simulink model "backstepping_compliant_two_motors"  (R2022b)
settings: Solver=VariableStepAuto  StartTime=0.0  StopTime=20  RelTol=1e-3
values from neighbouring files (symbols this model uses):
  Lamda = 1*eye(2)    [init.m]
undefined symbols (not defined in the file or in its folder): D, J
settings Model: Creator=alexi  LastModifiedBy=alexi

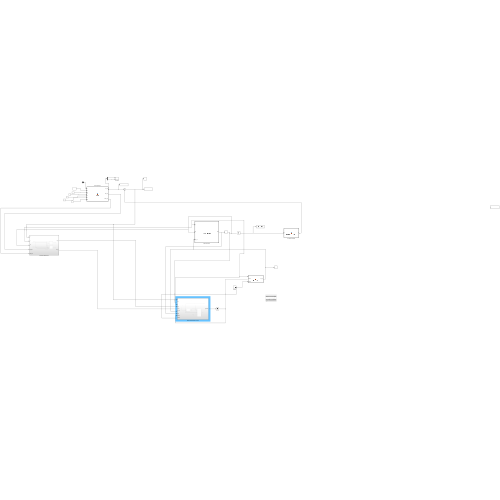
[thumbnail: Simulink's stored preview of the top-level diagram]
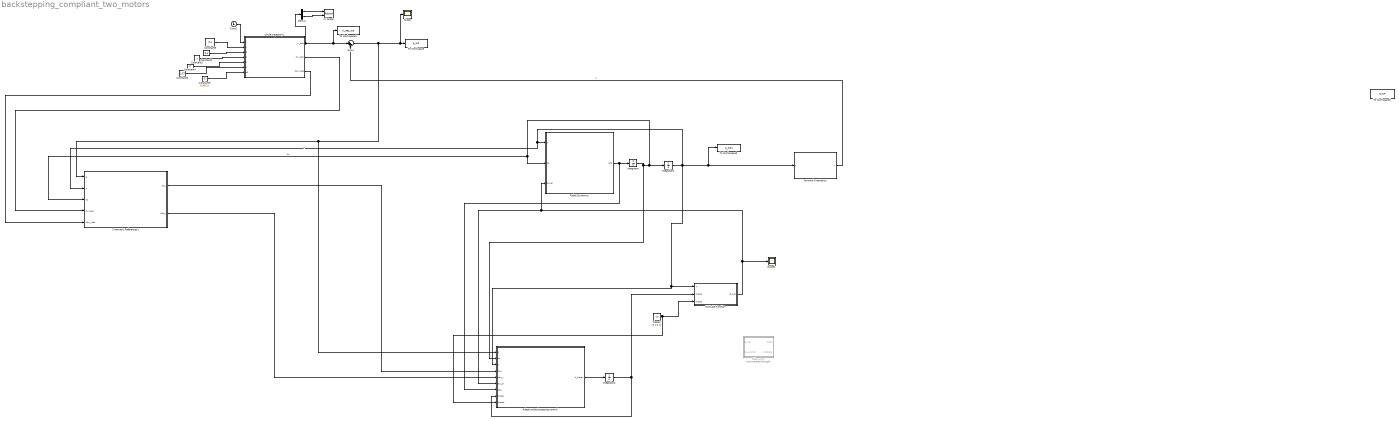
== system backstepping_compliant_two_motors ==
  Adaptive Backstepping control : Subsystem
  Clock1 : Clock
  Constant2 : Constant  Value=0.4
  Constant3 : Constant
  Constant4 : Constant  Value=2
  Constant5 : Constant  Value=1.57
  Constant6 : Constant  Value=[0.85,1]
  Constant9 : Constant  Value=0.4
  Demux : Demux  Outputs=2
  Forward Kinematics : MATLAB Function  TreatAsAtomicUnit=on
  Integrator : Integrator  InitialCondition=[0,0]'
  Integrator1 : Integrator  InitialCondition=[0.1,0.1]'
  Integrator2 : Integrator  InitialCondition=[0.1,0.1]'
  Kinematic References1 : Subsystem
  MATLAB Function : MATLAB Function  TreatAsAtomicUnit=on
  Robot Dynamics : MATLAB Function  TreatAsAtomicUnit=on
  Scope : Scope
  Scope1 : Scope
  Subsystem : Subsystem  Commented=through
  Sum4 : Sum  Inputs=|+-
  To Workspace : ToWorkspace  VariableName=e_out  SaveFormat=Timeseries  SampleTime=-1
  To Workspace1 : ToWorkspace  VariableName=xi_des_out  SaveFormat=Timeseries  SampleTime=-1
  To Workspace2 : ToWorkspace  VariableName=q_out  SaveFormat=Timeseries  SampleTime=-1
  To Workspace3 : ToWorkspace  VariableName=q_out1  SaveFormat=Timeseries  SampleTime=-1
  XY Graph : Record  FileSettingsInternal="{\"entries\":[{\"content\":{\"excelSettings\":{\"content\":{},\"type\":\"Streamout.ExcelSettings\"}},\"type\":\"Streamout.FileSettingStorage\",\"uuid\":\"296eadd8-438a-48ea-aa87-085f53f925dc\"}],\"packageUris\":[\"http://schema.mathworks.com/mf0/streamout_blocks/R2020a\"],\"version\":\"1.0\"}"  Layout=[1 1]  SignalsInternal="{\"entries\":[{\"content\":{\"signals\":[{\"content\":{\"blockPath\":[\"backstepping_compliant_two_motors/XY Graph\"],\"channel\":[],\"dimensions\":[1],\"domain\":\"backstepping_compliant_two_motors/XY Graph\",\"lineColor\":\"#a2142f\",\"plots\":[],\"port\":1,\"sid\":[\"\"],\"signalID\":2831,\"signalName\":\"Demux:1\"},\"type\":\"RecordBlkView.Signal\",\"uuid\":\"da436bb7-b6f0-4922-b408-d20702b7c22f\"},{\"content\":{\"blockPath\":[\"backstepping_compliant_two_motors/XY Graph\"],\"channel\":[],\"dimensions\":[1],\"domain\":\"backstepping_compliant_two_motors/XY Graph\",\"lineColor\":\"#139fff\",\"plots\":[],\"port\":2,\"sid\":[\"\"],\"signalID\":2835,\"signalName\":\"Demux:2\"},\"type\":\"RecordBlkView.Signal\",\"uuid\":\"9bd5da55-d73b-4537-9ebd-c9d85c402df8\"}]},\"type\":\"RecordBlkView.InputSignals\",\"uuid\":\"734fe5a4-c58d-4aeb-987a-d06effc65ad3\"}],\"packageUris\":[\"http://schema.mathworks.com/mf0/streamout_blocks/R2020a\"],\"version\":\"1.0\"}"  VisualizationBindings="{\"xyplotplugin\":{\"info\":[{\"series\":[],\"subplotID\":1}]}}"  CompatibilityTag=XY
  circle trajectory1 : MATLAB Function  TreatAsAtomicUnit=on
  thetad : Constant  Value=[0.1,0.1]'
  wires:
  Clock1/1 -> circle trajectory1/1(t)
  Constant9/1 -> circle trajectory1/2(A)
  Constant2/1 -> circle trajectory1/3(B)
  Constant3/1 -> circle trajectory1/4(a)
  Constant4/1 -> circle trajectory1/5(b)
  Constant5/1 -> circle trajectory1/6(d)
  Constant6/1 -> circle trajectory1/7(p0)
  Integrator/1 -> Adaptive Backstepping control/2(dq), Integrator1/1, Robot Dynamics/2(dq), Kinematic References1/3(dq)  "dq"
  Robot Dynamics/1(ddq) -> Adaptive Backstepping control/7(ddq), Integrator/1
  Integrator1/1 -> Adaptive Backstepping control/3(q), MATLAB Function/1(q), Forward Kinematics/1(q), To Workspace3/1, Kinematic References1/2(q), Robot Dynamics/1(q)  "q"
  circle trajectory1/1(xi_des) -> Demux/1, To Workspace1/1, Sum4/1
  Forward Kinematics/1(xi) -> Sum4/2  "xi"
  Sum4/1 -> Scope/1, To Workspace/1, Adaptive Backstepping control/1(e), Kinematic References1/1(e)
  circle trajectory1/2(dxi_des) -> Kinematic References1/4(dxi_des)
  Kinematic References1/1(dq_r) -> Adaptive Backstepping control/4(dq_r)
  Kinematic References1/2(ddq_r) -> Adaptive Backstepping control/5(ddq_r)
  Adaptive Backstepping control/1(d_thetas) -> Integrator2/1
  Integrator2/1 -> Adaptive Backstepping control/8(thetas), MATLAB Function/2(thetas)
  MATLAB Function/1(tau_el) -> Scope1/1, Robot Dynamics/3(tau_el), Adaptive Backstepping control/6(tau_el)
  circle trajectory1/3(ddxi_des) -> Kinematic References1/5(ddxi_des)
  Demux/1 -> XY Graph/1
  Demux/2 -> XY Graph/2
  thetad/1 -> Adaptive Backstepping control/9(thetad), MATLAB Function/3(thetad)

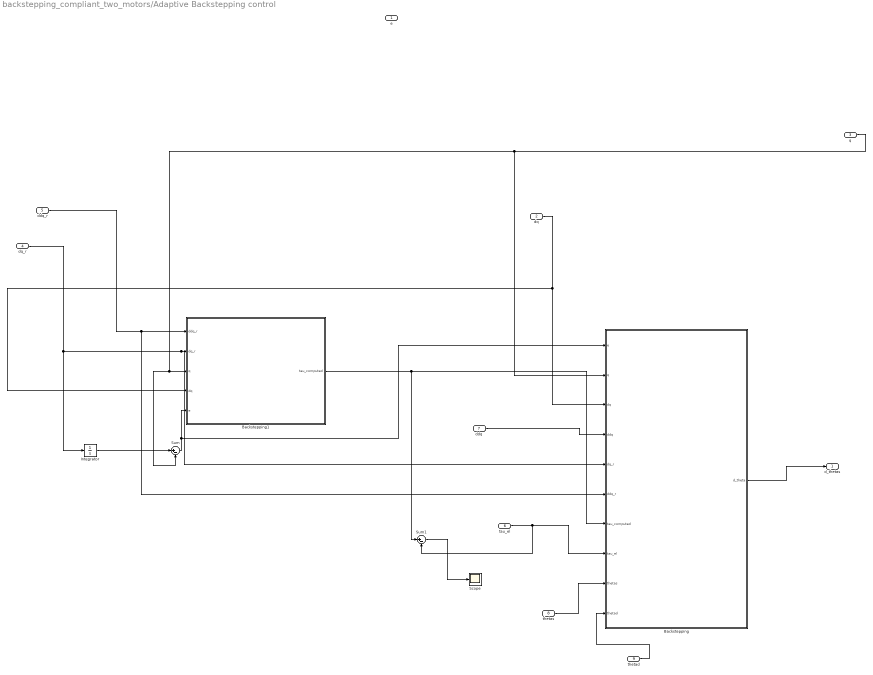
== system backstepping_compliant_two_motors/Adaptive Backstepping control ==
  e : Inport
  dq : Inport  Port=2
  q : Inport  Port=3
  dq_r : Inport  Port=4
  ddq_r : Inport  Port=5
  tau_el : Inport  Port=6
  ddq : Inport  Port=7
  thetas : Inport  Port=8
  thetad : Inport  Port=9
  Backstepping : MATLAB Function  TreatAsAtomicUnit=on
  Backstepping1 : MATLAB Function  TreatAsAtomicUnit=on
  Integrator : Integrator  InitialCondition=[0.1,0.1]'
  Scope : Scope
  Sum : Sum  Inputs=|+-
  Sum1 : Sum  Inputs=|+-
  d_thetas : Outport
  wires:
  dq_r/1 -> Integrator/1, Backstepping1/2(dq_r), Backstepping/5(dq_r)
  q/1 -> Backstepping/2(q), Backstepping1/3(q), Sum/2
  Backstepping1/1(tau_computed) -> Sum1/1, Backstepping/7(tau_computed)
  tau_el/1 -> Sum1/2, Backstepping/8(tau_el)
  ddq_r/1 -> Backstepping/6(ddq_r), Backstepping1/1(ddq_r)
  dq/1 -> Backstepping1/4(dq), Backstepping/3(dq)
  Backstepping/1(d_theta) -> d_thetas/1
  ddq/1 -> Backstepping/4(ddq)
  thetas/1 -> Backstepping/9(thetas)
  Integrator/1 -> Sum/1
  Sum/1 -> Backstepping1/5(e), Backstepping/1(e)
  thetad/1 -> Backstepping/10(thetad)
  Sum1/1 -> Scope/1

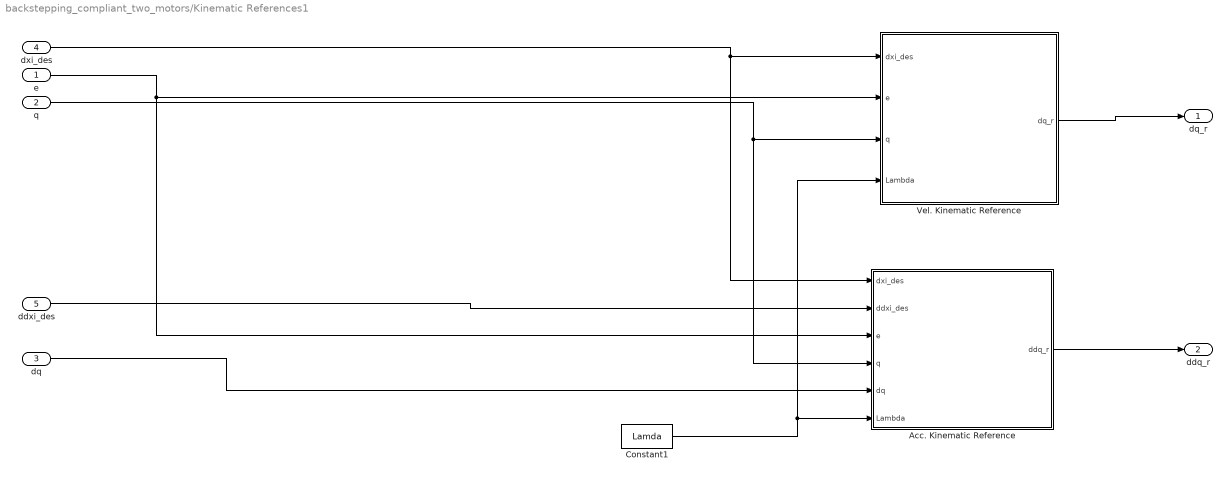
== system backstepping_compliant_two_motors/Kinematic References1 ==
  e : Inport
  q : Inport  Port=2
  dq : Inport  Port=3
  dxi_des : Inport  Port=4
  ddxi_des : Inport  Port=5
  Acc. Kinematic Reference : MATLAB Function  TreatAsAtomicUnit=on
  Constant1 : Constant  Value=Lamda
  "Vel. Kinematic Reference " : MATLAB Function  TreatAsAtomicUnit=on
  dq_r : Outport  VectorParamsAs1DForOutWhenUnconnected=off
  ddq_r : Outport  Port=2  VectorParamsAs1DForOutWhenUnconnected=off
  wires:
  ddxi_des/1 -> Acc. Kinematic Reference/2(ddxi_des)
  e/1 -> Acc. Kinematic Reference/3(e), "Vel. Kinematic Reference "/2(e)
  dxi_des/1 -> Acc. Kinematic Reference/1(dxi_des), "Vel. Kinematic Reference "/1(dxi_des)
  Constant1/1 -> "Vel. Kinematic Reference "/4(Lambda), Acc. Kinematic Reference/6(Lambda)
  "Vel. Kinematic Reference "/1(dq_r) -> dq_r/1
  dq/1 -> Acc. Kinematic Reference/5(dq)
  q/1 -> Acc. Kinematic Reference/4(q), "Vel. Kinematic Reference "/3(q)
  Acc. Kinematic Reference/1(ddq_r) -> ddq_r/1

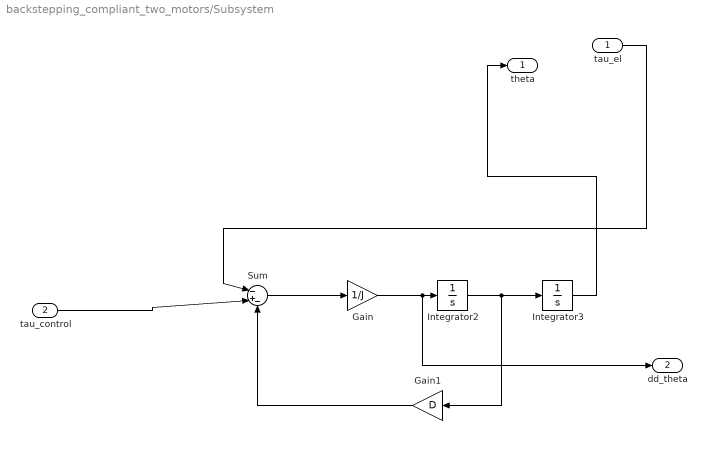
== system backstepping_compliant_two_motors/Subsystem ==
  tau_el : Inport
  tau_control : Inport  Port=2
  Gain : Gain  Gain=1/J
  Gain1 : Gain  Gain=D
  Integrator2 : Integrator
  Integrator3 : Integrator
  Sum : Sum  Inputs=|-+-
  theta : Outport
  dd_theta : Outport  Port=2
  wires:
  tau_control/1 -> Sum/2
  Integrator3/1 -> theta/1
  Integrator2/1 -> Gain1/1, Integrator3/1
  Gain1/1 -> Sum/3
  Gain/1 -> dd_theta/1, Integrator2/1
  Sum/1 -> Gain/1
  tau_el/1 -> Sum/1

== matlab function backstepping_compliant_two_motors/Kinematic References1/Acc. Kinematic Reference ==
  data: dxi_des input; ddq_r output; ddxi_des input; e input; q input; dq input; Lambda input
function ddq_r = acc_kinematic_reference(dxi_des, ddxi_des, e, q, dq, Lambda)

coder.extrinsic('disp');

J = zeros(2,2);
dJ = zeros(2,2);

dq1 = dq(1);
dq2 = dq(2);

q1 = q(1);
q2 = q(2);

a1 = 1;
a2 = 1;

% Computing jacobian and derivative
J = [-a2*sin(q1 + q2) - a1*sin(q1), -a2*sin(q1 + q2);
      a2*cos(q1 + q2) + a1*cos(q1),  a2*cos(q1 + q2)];

dJ = [-a2*cos(q1 + q2)*(dq1 + dq2)-a1*cos(q1)*dq1, -a2*cos(q1 + q2)*(dq1 + dq2);
    -a2*sin(q1 + q2)*(dq1 + dq2)-a1*sin(q1)*dq1, -a2*sin(q1 + q2)*(dq1 + dq2)];

ddq_r = inv(J) * (ddxi_des + Lambda*dxi_des - Lambda*J*dq) ...
- inv(J)*dJ*inv(J)*(dxi_des + Lambda*e);
end

== matlab function backstepping_compliant_two_motors/Kinematic References1/Vel. Kinematic Reference  ==
  data: dxi_des input; dq_r output; e input; q input; Lambda input
function dq_r = vel_kinematic_reference(dxi_des, e, q, Lambda)
a1 = 1;
a2 = 1;

q1 = q(1);
q2 = q(2);

% Computing jacobian
J = [-a2*sin(q1 + q2) - a1*sin(q1), -a2*sin(q1 + q2);
      a2*cos(q1 + q2) + a1*cos(q1),  a2*cos(q1 + q2)];

dq_r = inv(J) * (dxi_des + Lambda*e);
end

== matlab function backstepping_compliant_two_motors/Adaptive Backstepping control/Backstepping1 ==
  data: ddq_r input; dq_r input; q input; dq input; e input; tau_computed output
function tau_computed  = computed_torque(ddq_r,dq_r,q,dq,e)

coder.extrinsic('disp');
rel_err = 0;

de = dq_r-dq;
Kp = 35;
Kv = 12;

% Get dynamic matrices
B = RR_mass_matrix(q);
C = RR_coriolis_matrix(q,dq);
G = RR_gravity_vector(q);

% Adding uncertainty
B = B.*(1 + rel_err);
C = C.*(1 + rel_err);
G = G.*(1 + rel_err);

% Control law
tau_computed = -(B*ddq_r+C*dq+G+B*Kp*e+B*Kv*de);

== matlab function backstepping_compliant_two_motors/circle trajectory1 ==
  data: t input; xi_des output; dxi_des output; A input; B input; a input; b input; d input; p0 input; ddxi_des output
function [xi_des, dxi_des, ddxi_des] = lissajous(t,A,B,a,b,d,p0)

xi_des = [A*sin(a*t+d); B*sin(b*t)] + p0;
dxi_des = [A*a*cos(a*t+d); B*b*cos(b*t)];
ddxi_des = [-A*a^2*sin(a*t+d); -B*b^2*sin(b*t)];

== matlab function backstepping_compliant_two_motors/MATLAB Function ==
  data: q input; tau_el output; thetas input; thetad input
function tau_el = tau_elastica(q,thetas,thetad)
% k = 0.1;
% a = 9;
% k1_hat = pi(1);
% k2_hat = pi(2);
% k3_hat = pi(3);
% k4_hat = pi(4);
k1 = 100;
k2 = 100;
k3 = 100;
k4 = 100;

tau_el1 = k1*(q(1)-thetas(1)-thetad(1)) + k1*(q(1) - thetas(1) + thetad(1)) + k2*(q(1)-thetas(1) - thetad(1))^2 + k2*(q(1)-thetas(1) + thetad(1))^2 + k3*(q(1)-thetas(1) - thetad(1))^3 + k3*(q(1)-thetas(1) + thetad(1))^3 + k4*(q(1)-thetas(1) - thetad(1))^4 + k4*(q(1)-thetas(1) + thetad(1))^4;
tau_el2 = k1*(q(2)-thetas(2)-thetad(2)) + k1*(q(2) - thetas(2) + thetad(2)) + k2*(q(2)-thetas(2) - thetad(2))^2 + k2*(q(2)-thetas(2) + thetad(2))^2 + k3*(q(2)-thetas(2) - thetad(2))^3 + k3*(q(2)-thetas(2) + thetad(2))^3 + k4*(q(2)-thetas(2) - thetad(2))^4 + k4*(q(2)-thetas(2) + thetad(2))^4;
tau_el = [tau_el1;tau_el2];

== matlab function backstepping_compliant_two_motors/Adaptive Backstepping control/Backstepping ==
  data: e input; q input; dq input; ddq input; dq_r input; ddq_r input; tau_computed input; d_theta output; tau_el input; thetas input; thetad input
function d_theta  = backstepping(e,q,dq,ddq,dq_r,ddq_r,tau_computed,tau_el,thetas,thetad)

coder.extrinsic('disp');
rel_err = 0;
de = dq_r-dq;
dde = ddq_r-ddq;
P = 10*eye(2);
K = 0.1;
Kc = 100;
Kp = 35;
Kv = 12;
a = 9;
% k1_hat = 50;
% k2_hat = 50;
% k3_hat = 50;
% k4_hat = 50;
k1 = 100;
k2 = 100;
k3 = 100;
k4 = 100;

% Get dynamic matrices
B = RR_mass_matrix(q);
C = RR_coriolis_matrix(q,dq);
G = RR_gravity_vector(q);

% Adding uncertainty
B = B.*(1 + rel_err);
C = C.*(1 + rel_err);
G = G.*(1 + rel_err);
g = [zeros(2,2); pinv(B)];
d_tau = C*dde-B*Kv*dde-B*Kp*de;

a1 = 1;
a2 = 1;



% Control law
%d_theta = B*ddq_r + C*dq_r + G + Ks*de + J.'*e;
Vx1 = [e'*Kp,de'];

l1 = -k1 - k1 - 2*k2*(q(1)-thetas(1)-thetad(1)) - 2*k2*(q(1)-thetas(1) + thetad(1)) - 3*k3*(q(1)-thetas(1)-thetad(1))^2 - 3*k3*(q(1)-thetas(1)+thetad(1))^2 - 4*k4*(q(1)-thetas(1)-thetad(1))^3 - 4*k4*(q(1)-thetas(1)+thetad(1))^3 ;
l2 = -k1 - k1 - 2*k2*(q(2)-thetas(2)-thetad(2)) - 2*k2*(q(2)-thetas(2) + thetad(2)) - 3*k3*(q(2)-thetas(2)-thetad(2))^2 - 3*k3*(q(2)-thetas(2)+thetad(2))^2 - 4*k4*(q(2)-thetas(2)-thetad(2))^3 - 4*k4*(q(2)-thetas(2)+thetad(2))^3;


l = [l1 0; 0 l2];


h1 = k1*dq(1) + k1*dq(1) + 2*k2*(q(1)-thetas(1)-thetad(1))*dq(1) + 2*k2*(q(1)-thetas(1)+thetad(1))*dq(1) + 3*k3*dq(1)*(q(1)-thetas(1)-thetad(1))^2 + 3*k3*dq(1)*(q(1)-thetas(1)+thetad(1))^2 + 4*k4*dq(1)*(q(1)-thetas(1)-thetad(1))^3 + 4*k4*dq(1)*(q(1)-thetas(1)+thetad(1))^3;
h2 = k1*dq(2) + k1*dq(2) + 2*k2*(q(2)-thetas(2)-thetad(2))*dq(2) + 2*k2*(q(2)-thetas(2)+thetad(2))*dq(2) + 3*k3*dq(2)*(q(2)-thetas(2)-thetad(2))^2 + 3*k3*dq(2)*(q(2)-thetas(2)+thetad(2))^2 + 4*k4*dq(2)*(q(2)-thetas(2)-thetad(2))^3 + 4*k4*dq(2)*(q(2)-thetas(2)+thetad(2))^3;;

h = [h1;h2];

v = d_tau+pinv(P)*(Kc*(tau_computed-tau_el)-g'*Vx1');
d_theta = inv(l)*(v-h);

== matlab function backstepping_compliant_two_motors/Robot Dynamics ==
  data: q input; dq input; tau_el input; ddq output
function ddq = inverse_dynamics(q,dq, tau_el)

% Get dynamic matrices
B = RR_mass_matrix(q);
C = RR_coriolis_matrix(q,dq);
G = RR_gravity_vector(q);
ddq = pinv(B)*(-tau_el - C*dq - G);

== matlab function backstepping_compliant_two_motors/Forward Kinematics ==
  data: q input; xi output
function xi  = RR_forward_kinematics(q)

    q1 = q(1);
    q2 = q(2);

    a1 = 1;
    a2 = 1;

    p0 = [0;0];
    p1 = [a1*cos(q1); a1*sin(q1)];
    xi = p1+[a2*cos(q1+q2);a2*sin(q1+q2)];
end
